simulink model "Mando"  (R2017b)
settings: Solver=VariableStepDiscrete  StartTime=0.0  StopTime=inf  MaxStep=1e-4  RelTol=1e-3  EnableMultiTasking=on
libraries: vrlib x1, simulink x1, powerlib x1
settings Model: Creator=salas  LastModifiedBy=TrendingPC
settings OptimizationCC: LifeSpan=inf
settings DebuggingCC: SFUnexpectedBacktrackingDiag=warning  SFNoUnconditionalDefaultTransitionDiag=warning  SFExecutionAtInitializationDiag=none
settings CodeAppCC: StateflowObjectComments=on
settings GRTTargetCC: TargetLangStandard=C89/C90 (ANSI)  GeneratePreprocessorConditionals=Disable all
settings ConfigComp: CovMetricSettings=dw  CovHtmlReporting=on  CovSaveCumulativeToWorkspaceVar=on  CovSaveSingleToWorkspaceVar=on  CovExternalEMLEnable=off
settings SimscapeCC: SimscapeNormalizeSystem=off

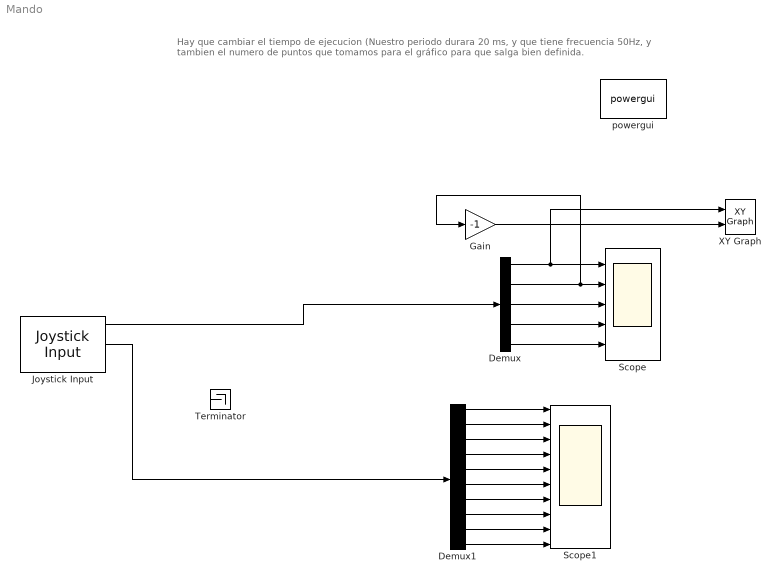
== system Mando ==
  note: Hay que cambiar el tiempo de ejecucion (Nuestro periodo durara 20 ms, y que tiene frecuencia 50Hz, y tambien el numero de puntos que tomamos para el gráfico para que salga bien definida.
  Demux : Demux  Outputs=5
  Demux1 : Demux  Outputs=10
  Gain : Gain  Gain=-1
  Joystick Input : vrlib/Joystick Input  joyid=1  adjustports=on  forcefeed=off
      settings: SourceProductBaseCode=VR
  Scope : Scope  NumInputPorts=5
  Scope1 : Scope  NumInputPorts=10
  Terminator : Terminator
  XY Graph : simulink/Sinks/XY Graph  xmin=-1  xmax=1  ymin=-1  ymax=1  st=-1
  powergui : powerlib/powergui  Priority=1  SimulationMode=Discrete  SampleTime=0.001  frequency=60  Iterations=50  frequencyindice=50  Pbase=100e6  ErrMax=1e-4  UnitsV=kV  UnitsW=MW  buscounter=0  FunctionMessages=off  echomessages=off  EnableUseOfTLC=off  CurrentSourceSwitches=off  DisableSnubberDevices=off  DisableRonSwitches=off  DisableVfSwitches=off  DisplayEquations=off  SolverType=Tustin/Backward Euler (TBE)  Interpol=off  ExternalGateDelay=off  methode=off  Ts=100  x0status=blocks  SPID=on  SwTol=0  HookPort=off  RestoreLinks=warning  ResistiveCurrentMeasurement=off  Frange=[0:2:500]  Ylog=off  Xlog=on  ShowGrid=off  save=off  variable=ZData  structure=0  ZoomFFT=off  StartTime=0.0  cycles=1  DisplayStyle=1  fundamental=60  FreqAxis=off  MaxFrequency=1000  frequencyindicesteady=1  RmsSteady=1  display=off
  wires:
  Joystick Input/1 -> Demux/1
  Demux/1 -> XY Graph/1, Scope/1
  Demux/3 -> Scope/3
  Demux/4 -> Scope/4
  Demux/5 -> Scope/5
  Gain/1 -> XY Graph/2
  Demux/2 -> Gain/1, Scope/2
  Demux1/1 -> Scope1/1
  Demux1/2 -> Scope1/2
  Demux1/3 -> Scope1/3
  Demux1/4 -> Scope1/4
  Demux1/5 -> Scope1/5
  Demux1/6 -> Scope1/6
  Demux1/7 -> Scope1/7
  Demux1/8 -> Scope1/8
  Demux1/9 -> Scope1/9
  Demux1/10 -> Scope1/10
  Joystick Input/2 -> Demux1/1
  ? -> Terminator/1
